simulink model "Architecture"  (R2025b)
settings: Solver=VariableStepAuto  StartTime=0.0  StopTime=10.0  RelTol=1e-3
settings Model: Creator=morit  LastModifiedBy=morit

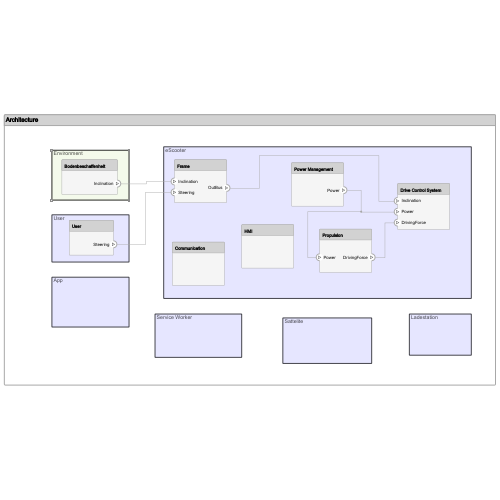
[thumbnail: Simulink's stored preview of the top-level diagram]
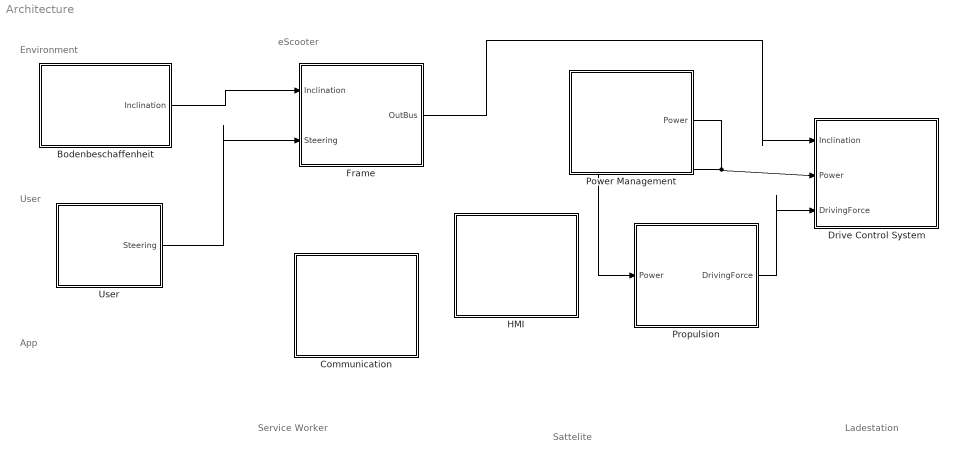
== system Architecture ==
  note: Sattelite
  note: Service Worker
  note: eScooter
  note: Ladestation
  note: User
  note: App
  note: Environment
  Bodenbeschaffenheit : Subsystem
      settings: PortSchema="{\"entries\":[{\"content\":{\"headerSize\":26,\"margin\":15,\"minimumSpacing\":25,\"sides\":[{\"content\":{},\"type\":\"ConnectorPlacement.EquallySpacedRectSide\",\"uuid\":\"dbaa959b-8c6e-4a4f-8fde-1e299d4bf125\"},{\"content\":{\"connectorIds\":[\"Out1\"],\"side\":\"RIGHT\"},\"type\":\"ConnectorPlacement.EquallySpacedRectSide\",\"uuid\":\"33a174a8-2572-4532-8d29-9e5235b9ab97\"},{\"content\":{\"side\":\"TOP\"},\"type\":\"ConnectorPlacement.EquallySpacedRectSide\",\"uuid\":\"7fa8e030-0ffa-41f9-8c39-892697cfd317\"}]},\"type\":\"ConnectorPlacement.EquallySpacedConnector\",\"uuid\":\"837daa9d-3923-43bf-8fcc-9a3bb0a11923\"}],\"packageUris\":[\"http://schema.mathworks.com/mf0/Connector/R2020b\"],\"version\":\"1.0\"}"
  Communication : Subsystem
      settings: PortSchema="{\"entries\":[{\"content\":{\"headerSize\":26,\"margin\":15,\"minimumSpacing\":25,\"sides\":[{\"content\":{},\"type\":\"ConnectorPlacement.EquallySpacedRectSide\",\"uuid\":\"dbaa959b-8c6e-4a4f-8fde-1e299d4bf125\"},{\"content\":{\"side\":\"RIGHT\"},\"type\":\"ConnectorPlacement.EquallySpacedRectSide\",\"uuid\":\"33a174a8-2572-4532-8d29-9e5235b9ab97\"},{\"content\":{\"side\":\"TOP\"},\"type\":\"ConnectorPlacement.EquallySpacedRectSide\",\"uuid\":\"7fa8e030-0ffa-41f9-8c39-892697cfd317\"}]},\"type\":\"ConnectorPlacement.EquallySpacedConnector\",\"uuid\":\"837daa9d-3923-43bf-8fcc-9a3bb0a11923\"}],\"packageUris\":[\"http://schema.mathworks.com/mf0/Connector/R2020b\"],\"version\":\"1.0\"}"
  Drive Control System : Subsystem
      settings: PortSchema="{\"entries\":[{\"content\":{\"headerSize\":26,\"margin\":15,\"minimumSpacing\":25,\"sides\":[{\"content\":{\"connectorIds\":[\"In1\",\"In2\",\"In3\"]},\"type\":\"ConnectorPlacement.EquallySpacedRectSide\",\"uuid\":\"dbaa959b-8c6e-4a4f-8fde-1e299d4bf125\"},{\"content\":{\"side\":\"RIGHT\"},\"type\":\"ConnectorPlacement.EquallySpacedRectSide\",\"uuid\":\"33a174a8-2572-4532-8d29-9e5235b9ab97\"},{\"content\":{\"side\":\"TOP\"},\"type\":\"ConnectorPlacement.EquallySpacedRectSide\",\"uuid\":\"7fa8e030-0ffa-41f9-8c39-892697cfd317\"}]},\"type\":\"ConnectorPlacement.EquallySpacedConnector\",\"uuid\":\"837daa9d-3923-43bf-8fcc-9a3bb0a11923\"}],\"packageUris\":[\"http://schema.mathworks.com/mf0/Connector/R2020b\"],\"version\":\"1.0\"}"
  Frame : Subsystem
      settings: PortSchema="{\"entries\":[{\"content\":{\"headerSize\":26,\"margin\":15,\"minimumSpacing\":25,\"sides\":[{\"content\":{\"connectorIds\":[\"In1\",\"In2\"]},\"type\":\"ConnectorPlacement.EquallySpacedRectSide\",\"uuid\":\"dbaa959b-8c6e-4a4f-8fde-1e299d4bf125\"},{\"content\":{\"connectorIds\":[\"Out1\"],\"side\":\"RIGHT\"},\"type\":\"ConnectorPlacement.EquallySpacedRectSide\",\"uuid\":\"33a174a8-2572-4532-8d29-9e5235b9ab97\"},{\"content\":{\"side\":\"TOP\"},\"type\":\"ConnectorPlacement.EquallySpacedRectSide\",\"uuid\":\"7fa8e030-0ffa-41f9-8c39-892697cfd317\"}]},\"type\":\"ConnectorPlacement.EquallySpacedConnector\",\"uuid\":\"837daa9d-3923-43bf-8fcc-9a3bb0a11923\"}],\"packageUris\":[\"http://schema.mathworks.com/mf0/Connector/R2020b\"],\"version\":\"1.0\"}"
  HMI : Subsystem
      settings: PortSchema="{\"entries\":[{\"content\":{\"headerSize\":26,\"margin\":15,\"minimumSpacing\":25,\"sides\":[{\"content\":{},\"type\":\"ConnectorPlacement.EquallySpacedRectSide\",\"uuid\":\"dbaa959b-8c6e-4a4f-8fde-1e299d4bf125\"},{\"content\":{\"side\":\"RIGHT\"},\"type\":\"ConnectorPlacement.EquallySpacedRectSide\",\"uuid\":\"33a174a8-2572-4532-8d29-9e5235b9ab97\"},{\"content\":{\"side\":\"TOP\"},\"type\":\"ConnectorPlacement.EquallySpacedRectSide\",\"uuid\":\"7fa8e030-0ffa-41f9-8c39-892697cfd317\"}]},\"type\":\"ConnectorPlacement.EquallySpacedConnector\",\"uuid\":\"837daa9d-3923-43bf-8fcc-9a3bb0a11923\"}],\"packageUris\":[\"http://schema.mathworks.com/mf0/Connector/R2020b\"],\"version\":\"1.0\"}"
  Power Management : Subsystem
      settings: PortSchema="{\"entries\":[{\"content\":{\"headerSize\":26,\"margin\":15,\"minimumSpacing\":25,\"sides\":[{\"content\":{},\"type\":\"ConnectorPlacement.EquallySpacedRectSide\",\"uuid\":\"dbaa959b-8c6e-4a4f-8fde-1e299d4bf125\"},{\"content\":{\"connectorIds\":[\"Out1\"],\"side\":\"RIGHT\"},\"type\":\"ConnectorPlacement.EquallySpacedRectSide\",\"uuid\":\"33a174a8-2572-4532-8d29-9e5235b9ab97\"},{\"content\":{\"side\":\"TOP\"},\"type\":\"ConnectorPlacement.EquallySpacedRectSide\",\"uuid\":\"7fa8e030-0ffa-41f9-8c39-892697cfd317\"}]},\"type\":\"ConnectorPlacement.EquallySpacedConnector\",\"uuid\":\"837daa9d-3923-43bf-8fcc-9a3bb0a11923\"}],\"packageUris\":[\"http://schema.mathworks.com/mf0/Connector/R2020b\"],\"version\":\"1.0\"}"
  Propulsion : Subsystem
      settings: PortSchema="{\"entries\":[{\"content\":{\"headerSize\":26,\"margin\":15,\"minimumSpacing\":25,\"sides\":[{\"content\":{\"connectorIds\":[\"In1\"]},\"type\":\"ConnectorPlacement.EquallySpacedRectSide\",\"uuid\":\"dbaa959b-8c6e-4a4f-8fde-1e299d4bf125\"},{\"content\":{\"connectorIds\":[\"Out1\"],\"side\":\"RIGHT\"},\"type\":\"ConnectorPlacement.EquallySpacedRectSide\",\"uuid\":\"33a174a8-2572-4532-8d29-9e5235b9ab97\"},{\"content\":{\"side\":\"TOP\"},\"type\":\"ConnectorPlacement.EquallySpacedRectSide\",\"uuid\":\"7fa8e030-0ffa-41f9-8c39-892697cfd317\"}]},\"type\":\"ConnectorPlacement.EquallySpacedConnector\",\"uuid\":\"837daa9d-3923-43bf-8fcc-9a3bb0a11923\"}],\"packageUris\":[\"http://schema.mathworks.com/mf0/Connector/R2020b\"],\"version\":\"1.0\"}"
  User : Subsystem
      settings: PortSchema="{\"entries\":[{\"content\":{\"headerSize\":26,\"margin\":15,\"minimumSpacing\":25,\"sides\":[{\"content\":{},\"type\":\"ConnectorPlacement.EquallySpacedRectSide\",\"uuid\":\"dbaa959b-8c6e-4a4f-8fde-1e299d4bf125\"},{\"content\":{\"connectorIds\":[\"Out1\"],\"side\":\"RIGHT\"},\"type\":\"ConnectorPlacement.EquallySpacedRectSide\",\"uuid\":\"33a174a8-2572-4532-8d29-9e5235b9ab97\"},{\"content\":{\"side\":\"TOP\"},\"type\":\"ConnectorPlacement.EquallySpacedRectSide\",\"uuid\":\"7fa8e030-0ffa-41f9-8c39-892697cfd317\"}]},\"type\":\"ConnectorPlacement.EquallySpacedConnector\",\"uuid\":\"837daa9d-3923-43bf-8fcc-9a3bb0a11923\"}],\"packageUris\":[\"http://schema.mathworks.com/mf0/Connector/R2020b\"],\"version\":\"1.0\"}"
  wires:
  Bodenbeschaffenheit/1(Inclination) -> Frame/1(Inclination)
  Power Management/1(Power) -> Propulsion/1(Power), Drive Control System/2(Power)
  Propulsion/1(DrivingForce) -> Drive Control System/3(DrivingForce)
  Frame/1(OutBus) -> Drive Control System/1(Inclination)
  User/1(Steering) -> Frame/2(Steering)

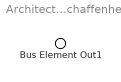
== system Architecture/Bodenbeschaffenheit ==
  Bus Element Out1 : Outport  PortName=Inclination

== system Architecture/Communication ==

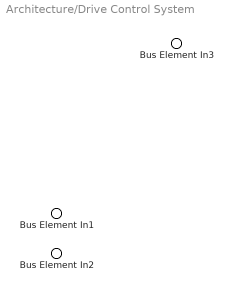
== system Architecture/Drive Control System ==
  Bus Element In3 : Inport  PortName=Inclination
  Bus Element In1 : Inport  Port=2  PortName=Power
  Bus Element In2 : Inport  Port=3  PortName=DrivingForce

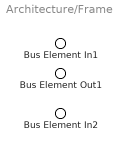
== system Architecture/Frame ==
  Bus Element In1 : Inport  PortName=Inclination
  Bus Element In2 : Inport  Port=2  PortName=Steering
  Bus Element Out1 : Outport  PortName=OutBus

== system Architecture/HMI ==

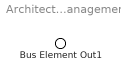
== system Architecture/Power Management ==
  Bus Element Out1 : Outport  PortName=Power

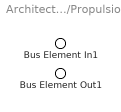
== system Architecture/Propulsion ==
  Bus Element In1 : Inport  PortName=Power
  Bus Element Out1 : Outport  PortName=DrivingForce

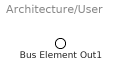
== system Architecture/User ==
  Bus Element Out1 : Outport  PortName=Steering
